simulink model "product"  (R2015a)
settings: Solver=ode45  StartTime=0.0  StopTime=1000.0  RelTol=1e-3
values from neighbouring files (symbols this model uses):
  alpha_const = 0.0    (= 0)    [averagedRelayOutput.m]    (also in bursting_linearised.m = 0.1; fastSlow.m; manParamsNullclines.m; manipulateParameters.m = getappdata(hObject.Parent,'alpha_const'))
  beta = 0.37    [averagedRelayOutput.m]    (also in bursting_linearised.m = 0.27; compareApproximations.m = 1.5; fastSlow.m; fast_nullcline_winged_cusp.m = 0.5)
  gamma = 0    [averagedRelayOutput.m]    (also in bursting_linearised.m = 1; compareApproximations.m = 1; fastSlow.m; fast_nullcline_winged_cusp.m = 1)
  slow_plant_X0 = -1.0    (= -1)    [averagedRelayOutput.m]    (also in bursting_linearised.m = -1.05; fastSlow.m; fast_nullcline_winged_cusp.m = -2; hRose.m = -10)
  ts = 1    [averagedRelayOutput.m]    (also in bursting_linearised.m; compareApproximations.m; fastSlow.m; fast_nullcline_winged_cusp.m)
  tus = 800    [averagedRelayOutput.m]    (also in bursting_linearised.m; fastSlow.m; manParamsNullclines.m; manipulateParameters.m = getappdata(hObject.Parent,'tus'))
  ultra_slow_plant_X0 = 0.45    [averagedRelayOutput.m]    (also in bursting_linearised.m = 0; fastSlow.m; hRose.m = 2000; manParamsNullclines.m)
settings Model: CovModelRefEnable=off  Creator=rajiv  LastModifiedBy=rajiv
settings DataIOCC: SaveFormat=Dataset
settings HardwareCC: ProdBitPerPointer=64  ProdLargestAtomicFloat=Float  ProdIntDivRoundTo=Zero  ProdEndianess=LittleEndian  ProdHWDeviceType=Specified
settings GRTTargetCC: GeneratePreprocessorConditionals=Use local settings

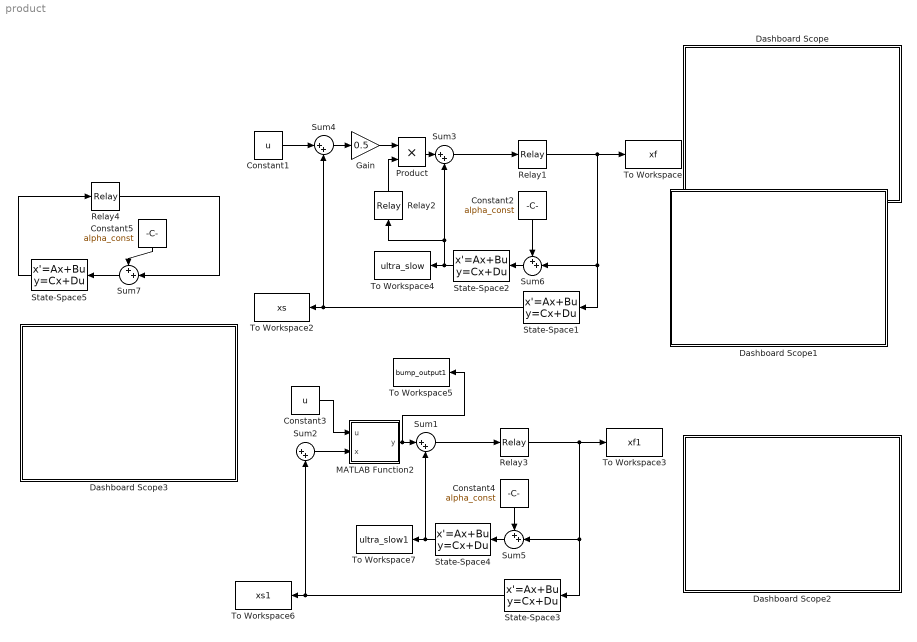
== system product ==
  Constant1 : Constant  Value=u
  Constant2 : Constant  Value=alpha_const
  Constant3 : Constant  Value=u
  Constant4 : Constant  Value=alpha_const
  Constant5 : Constant  Value=alpha_const
  Dashboard Scope : Subsystem  DialogController=hmiCreateDDGDialog  IsWebBlock=on  mask(MWDashboardBlock){webBlockId=b548e409-cc17-49aa-ad8a-10220872f5dc, webBlockType=sdiscope, ShowInitialText=on, HMISrcModelName=product}
      mask prompts: webBlockId "WebBlock Id"; webBlockType "WebBlock Type"; HMISrcModelName "Source Model"
      mask Help: helpview([docroot '/mapfiles/simulink.map'], 'hmi_scope')
      mask Display:
      | if strcmp(get_param(bdroot(gcb),'BlockDiagramType'), 'library')
      |     image([(matlabroot) '/toolbox/simulink/hmi/icons/DashboardScope.png']);
      | end
  Dashboard Scope1 : Subsystem  DialogController=hmiCreateDDGDialog  IsWebBlock=on  mask(MWDashboardBlock){webBlockId=1da811df-f941-4070-964f-177e56b51202, webBlockType=sdiscope, ShowInitialText=on, HMISrcModelName=product}
      mask prompts: webBlockId "WebBlock Id"; webBlockType "WebBlock Type"; HMISrcModelName "Source Model"
      mask Help: helpview([docroot '/mapfiles/simulink.map'], 'hmi_scope')
      mask Display:
      | if strcmp(get_param(bdroot(gcb),'BlockDiagramType'), 'library')
      |     image([(matlabroot) '/toolbox/simulink/hmi/icons/DashboardScope.png']);
      | end
  Dashboard Scope2 : Subsystem  DialogController=hmiCreateDDGDialog  IsWebBlock=on  mask(MWDashboardBlock){webBlockId=683791ea-ced5-4752-8832-f4de122e41d7, webBlockType=sdiscope, ShowInitialText=on, HMISrcModelName=product}
      mask prompts: webBlockId "WebBlock Id"; webBlockType "WebBlock Type"; HMISrcModelName "Source Model"
      mask Help: helpview([docroot '/mapfiles/simulink.map'], 'hmi_scope')
      mask Display:
      | if strcmp(get_param(bdroot(gcb),'BlockDiagramType'), 'library')
      |     image([(matlabroot) '/toolbox/simulink/hmi/icons/DashboardScope.png']);
      | end
  Dashboard Scope3 : Subsystem  DialogController=hmiCreateDDGDialog  IsWebBlock=on  mask(MWDashboardBlock){webBlockId=a9a41d6f-7146-4eb5-9415-6daf3ffd9162, webBlockType=sdiscope, ShowInitialText=on, HMISrcModelName=product}
      mask prompts: webBlockId "WebBlock Id"; webBlockType "WebBlock Type"; HMISrcModelName "Source Model"
      mask Help: helpview([docroot '/mapfiles/simulink.map'], 'hmi_scope')
      mask Display:
      | if strcmp(get_param(bdroot(gcb),'BlockDiagramType'), 'library')
      |     image([(matlabroot) '/toolbox/simulink/hmi/icons/DashboardScope.png']);
      | end
  Gain : Gain  Gain=0.5
  MATLAB Function2 : MATLAB Function  TreatAsAtomicUnit=on
      settings: PermitHierarchicalResolution=ParametersOnly
  Product : Product
  Relay1 : Relay  OnSwitchValue=beta  OffSwitchValue=-beta  OffOutputValue=-1
  Relay2 : Relay  OnSwitchValue=beta-0.5*(u-1/ts-0.5*gamma)  OffSwitchValue=beta  OnOutputValue=-1  OffOutputValue=1
  Relay3 : Relay  OnSwitchValue=beta  OffSwitchValue=-beta  OffOutputValue=-1
  Relay4 : Relay  OnSwitchValue=beta-0.5*(u-1/ts-0.5*gamma)  OffSwitchValue=beta  OnOutputValue=0  OffOutputValue=-1
  State-Space1 : StateSpace  A=-1/ts  B=1/ts  D=0.5*1*gamma  X0=slow_plant_X0
  State-Space2 : StateSpace  A=-1/tus  B=-1/tus  D=0  X0=ultra_slow_plant_X0
  State-Space3 : StateSpace  A=-1/ts  B=1/ts  D=0.5*1*gamma  X0=slow_plant_X0
  State-Space4 : StateSpace  A=-1/tus  B=-1/tus  D=0  X0=ultra_slow_plant_X0
  State-Space5 : StateSpace  A=-1/tus  B=-1/tus  D=0  X0=ultra_slow_plant_X0
  Sum{1..4} (4 alike) : Sum  Inputs=|++
  Sum5 : Sum  Inputs=++|
  Sum6 : Sum  Inputs=++|
  Sum7 : Sum  Inputs=++|
  To Workspace : ToWorkspace  VariableName=xf  SaveFormat=Timeseries  SampleTime=-1
  To Workspace2 : ToWorkspace  VariableName=xs  SaveFormat=Timeseries  SampleTime=-1
  To Workspace3 : ToWorkspace  VariableName=xf1  SaveFormat=Timeseries  SampleTime=-1
  To Workspace4 : ToWorkspace  VariableName=ultra_slow  SaveFormat=Timeseries  SampleTime=-1
  To Workspace5 : ToWorkspace  VariableName=bump_output1  SaveFormat=Timeseries  SampleTime=-1
  To Workspace6 : ToWorkspace  VariableName=xs1  SaveFormat=Timeseries  SampleTime=-1
  To Workspace7 : ToWorkspace  VariableName=ultra_slow1  SaveFormat=Timeseries  SampleTime=-1
  wires:
  Sum3/1 -> Relay1/1
  Constant1/1 -> Sum4/1
  Relay1/1 -> Sum6/2, State-Space1/1, To Workspace/1
  State-Space1/1 -> Sum4/2, To Workspace2/1
  Constant2/1 -> Sum6/1
  Sum6/1 -> State-Space2/1
  Sum4/1 -> Gain/1
  State-Space2/1 -> Sum3/2, Relay2/1, To Workspace4/1
  Gain/1 -> Product/1
  Product/1 -> Sum3/1
  Relay2/1 -> Product/2
  Sum1/1 -> Relay3/1
  Constant3/1 -> MATLAB Function2/1(u)
  Relay3/1 -> Sum5/2, State-Space3/1, To Workspace3/1
  State-Space3/1 -> Sum2/2, To Workspace6/1
  Constant4/1 -> Sum5/1
  Sum5/1 -> State-Space4/1
  Sum2/1 -> MATLAB Function2/2(x)
  MATLAB Function2/1(y) -> To Workspace5/1, Sum1/1
  State-Space4/1 -> To Workspace7/1, Sum1/2
  Constant5/1 -> Sum7/1
  Sum7/1 -> State-Space5/1
  Relay4/1 -> Sum7/2
  State-Space5/1 -> Relay4/1

== system product/Dashboard Scope ==

== system product/Dashboard Scope1 ==

== system product/Dashboard Scope2 ==

== system product/Dashboard Scope3 ==

== matlab function product/MATLAB Function2 ==
  data: u input; x input; y output
function y = fcn(u,x)
%#codegen
if (x < -2-u)
    y = -1;
elseif (x > 2-u)
    y = -1;
elseif and( x>=-2-u,x < -u)
    y = 0.5*(x+u);
else
    y = -0.5*(x+u);
end
